simulink model "sine"  (R2019b)
settings: Solver=VariableStepAuto  StartTime=0.0  StopTime=10.0  RelTol=1e-3
settings Model: Creator=Admin  LastModifiedBy=Admin

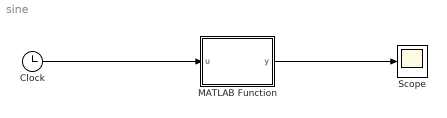
== system sine ==
  Clock : Clock
  MATLAB Function : MATLAB Function  TreatAsAtomicUnit=on
  Scope : Scope
  wires:
  Clock/1 -> MATLAB Function/1(u)
  MATLAB Function/1(y) -> Scope/1

== matlab function sine/MATLAB Function ==
  data: u input; y output
function y = sin(u)

y = sin(u);
